simulink model "firstOrderUnityNegativeFeedbackSystem"  (R2021b)
settings: Solver=VariableStepAuto  StartTime=0.0  StopTime=10.0  RelTol=1e-3
libraries: cstblocks x2
settings Model: Creator=PRANAV ARYA  LastModifiedBy=PRANAV ARYA

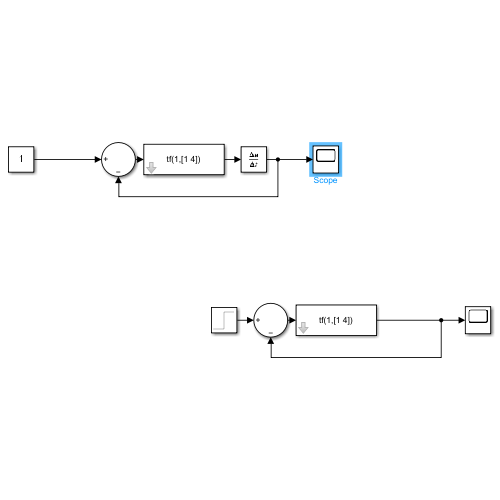
[thumbnail: Simulink's stored preview of the top-level diagram]
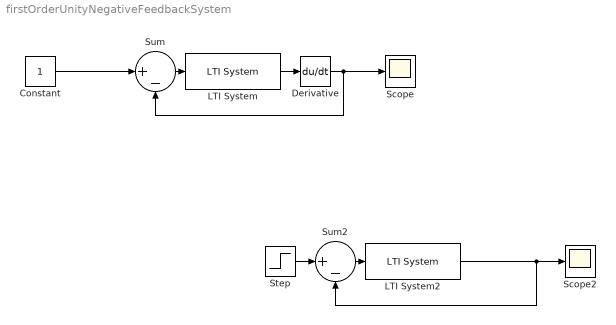
== system firstOrderUnityNegativeFeedbackSystem ==
  Constant : Constant
  Derivative : Derivative
  LTI System : cstblocks/LTI System  sys=tf(1,[1 4])  IC=[]
  LTI System2 : cstblocks/LTI System  sys=tf(1,[1 4])  IC=[]
  Scope : Scope
  Scope2 : Scope
  Step : Step  SampleTime=0
  Sum : Sum  Inputs=|+-
  Sum2 : Sum  Inputs=|+-
  wires:
  Sum/1 -> LTI System/1
  LTI System/1 -> Derivative/1
  Constant/1 -> Sum/1
  Derivative/1 -> Scope/1, Sum/2
  Sum2/1 -> LTI System2/1
  LTI System2/1 -> Sum2/2, Scope2/1
  Step/1 -> Sum2/1
